simulink model "simX_cosimulation"  (R2019b)
settings: Solver=VariableStepAuto  StartTime=0.0  StopTime=10.0  RelTol=1e-3
undefined symbols (not defined in the file): eta_0, eta_ref, thrust_lower_limit, thrust_upper_limit
libraries: simulink x1
settings Model: Creator=logan  LastModifiedBy=logan
settings OptimizationCC: UseDivisionForNetSlopeComputation=on

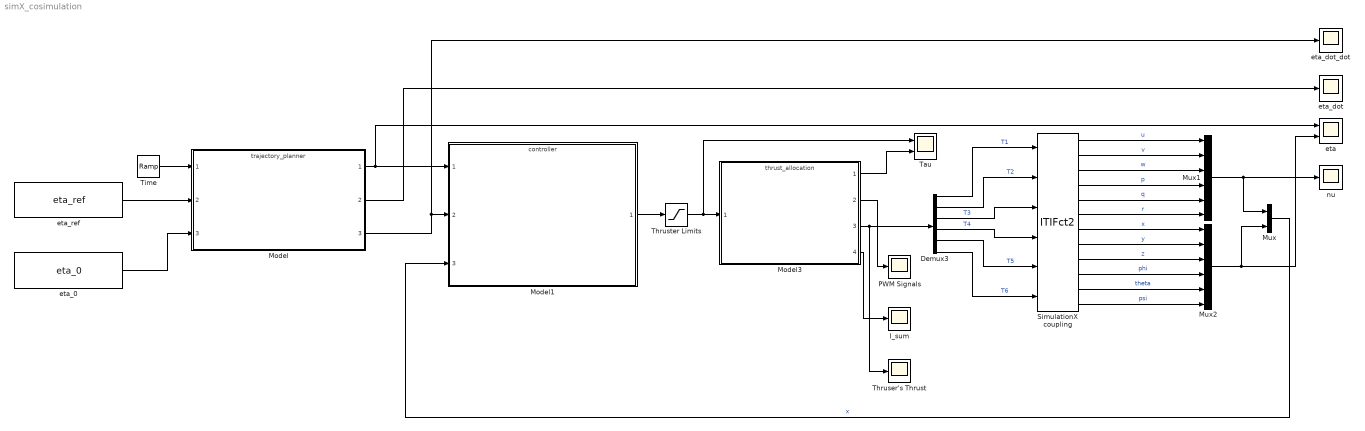
== system simX_cosimulation ==
  Demux3 : Demux  Outputs=6
  I_sum : Scope
  Model : ModelReference  ModelNameDialog=trajectory_planner.slx  SimulationMode=Normal  ModelReferenceVersion=1.26
  Model1 : ModelReference  ModelNameDialog=controller.slx  SimulationMode=Normal  ModelReferenceVersion=1.70
  Model3 : ModelReference  ModelNameDialog=thrust_allocation.slx  SimulationMode=Normal  ModelReferenceVersion=1.74
  Mux : Mux  Inputs=2
  Mux1 : Mux  Inputs=6
  Mux2 : Mux  Inputs=6
  PWM Signals : Scope
  SimulationX coupling : S-Function  FunctionName=ITIFct2  Parameters=ip, port, ts, nIn, nOut  SFunctionDeploymentMode=off  EnableBusSupport=off  mask{ip='localhost', port=4097, ts=0.001, nIn=6, nOut=12}
      mask prompts: ip "Address: ip"; port "Port Number: port [-]"; ts "Communication Step Size: ts [s]"; nIn "Input Vector Dimension (to SimulationX): nIn [-]"; nOut "Output Vector Dimension (from SimulationX): nOut [-]"
      mask help: Coupling Element
  Tau : Scope  NumInputPorts=2
  Thruser's Thrust : Scope
  Thruster Limits : Saturate  UpperLimit=thrust_upper_limit  LowerLimit=thrust_lower_limit
  "Time " : simulink/Sources/Ramp  slope=1  start=0  InitialOutput=0
  eta : Scope  NumInputPorts=2
  "eta_0 " : Constant  Value=eta_0
  eta_dot : Scope
  eta_dot_dot : Scope
  eta_ref : Constant  Value=eta_ref
  nu : Scope
  wires:
  SimulationX coupling/2 -> Mux1/2  "v"
  SimulationX coupling/12 -> Mux2/6  "psi"
  SimulationX coupling/5 -> Mux1/5  "q"
  SimulationX coupling/7 -> Mux2/1  "x"
  SimulationX coupling/11 -> Mux2/5  "theta"
  SimulationX coupling/10 -> Mux2/4  "phi"
  SimulationX coupling/9 -> Mux2/3  "z"
  Model3/1 -> Tau/2
  Demux3/5 -> SimulationX coupling/5  "T5"
  Demux3/3 -> SimulationX coupling/3  "T3"
  SimulationX coupling/1 -> Mux1/1  "u"
  SimulationX coupling/3 -> Mux1/3  "w"
  Demux3/1 -> SimulationX coupling/1  "T1"
  SimulationX coupling/4 -> Mux1/4  "p"
  Mux/1 -> Model1/3  "x"
  Model3/2 -> PWM Signals/1
  Demux3/6 -> SimulationX coupling/6  "T6"
  SimulationX coupling/6 -> Mux1/6  "r"
  SimulationX coupling/8 -> Mux2/2  "y"
  Model3/4 -> I_sum/1
  Model1/1 -> Thruster Limits/1
  Demux3/4 -> SimulationX coupling/4  "T4"
  Thruster Limits/1 -> Model3/1, Tau/1
  Model/3 -> Model1/2, eta_dot_dot/1
  eta_ref/1 -> Model/2
  Model3/3 -> Thruser's Thrust/1, Demux3/1
  Model/2 -> eta_dot/1
  "Time "/1 -> Model/1
  Demux3/2 -> SimulationX coupling/2  "T2"
  Model/1 -> Model1/1, eta/1
  Mux1/1 -> nu/1, Mux/1
  Mux2/1 -> Mux/2, eta/2
  "eta_0 "/1 -> Model/3
